simulink model "SG_RaibertControlMonopod"  (R2022a)
settings: Solver=ode4  StartTime=0.0  StopTime=inf  FixedStep=1/4000  MaxStep=0.001  RelTol=1e-3  AbsTol=1e-3  EnableMultiTasking=on
values from neighbouring files (symbols this model uses):
  alternate_legs = InitConstants.alternate_legs    [Controller.m]    (also in ControllerV2.m; ControllerV3.m; Controller_original.m; initialization.m = 1)
  dphi_IC = InitConstants.dphi_IC    [Controller.m]    (also in ControllerV2.m; ControllerV3.m; Controller_original.m; initialization.m = 0)
  dphi_RC_14 = 0.0    (= 0)    [initialization.m]
  dphi_RC_23 = 0.0    (= 0)    [initialization.m]
  dr_contact = -0.2    [initialization.m]
  dr_IC = InitConstants.dr_IC    [Controller.m]    (also in ControllerV2.m; ControllerV3.m; Controller_original.m; initialization.m = 0)
  dr_RC_14 = 0.0    (= 0)    [initialization.m]
  dr_RC_23 = 0.0    (= 0)    [initialization.m]
  dx_des = -InitConstants.dx_des    [Controller.m]    (also in ControllerV2.m; ControllerV3.m; Controller_original.m; Hopper_raibert_controller.m = -min(max(1.0*(x_body - x_des), -0.5), 0.5))
  Fthrust_RC_14 = 100    [initialization.m]
  Fthrust_RC_23 = 150    [initialization.m]
  GAIN_dx_RC_14 = 0.07    [initialization.m]
  GAIN_dx_RC_23 = 0.05    [initialization.m]
  Kd_phi_IC = InitConstants.Kd_phi_IC    [Controller.m]    (also in ControllerV2.m; ControllerV3.m; Controller_original.m; initialization.m = 15)
  Kd_phi_RC_14 = Kp_phi_RC_14*0.1    (= 10)    [initialization.m]
  Kd_phi_RC_23 = 15    [initialization.m]
  Kd_r_IC = InitConstants.Kd_r_IC    [Controller.m]    (also in ControllerV2.m; ControllerV3.m; Controller_original.m; initialization.m = 60)
  Kd_r_RC_14 = Kp_r_RC_14*0.1    (= 60)    [initialization.m]
  Kd_r_RC_23 = 150    [initialization.m]
  knee_limit = 160    [initialization.m]
  Kp_phi_IC = InitConstants.Kp_phi_IC    [Controller.m]    (also in ControllerV2.m; ControllerV3.m; Controller_original.m; initialization.m = 100)
  Kp_phi_RC_14 = 100    [initialization.m]
  Kp_phi_RC_23 = 100    [initialization.m]
  Kp_r_IC = InitConstants.Kp_r_IC    [Controller.m]    (also in ControllerV2.m; ControllerV3.m; Controller_original.m; initialization.m = 500)
  Kp_r_RC_14 = 600    [initialization.m]
  Kp_r_RC_23 = 600    [initialization.m]
  m_eff = 5    [ControllerV2.m]    (also in Controller_original.m; initialization.m)
  match_leg_gains = -1    [initialization.m]
  offset_phi_limit = 30    [initialization.m]
  phi_IC = InitConstants.phi_IC    [Controller.m]    (also in ControllerV2.m; ControllerV3.m; Controller_original.m; initialization.m = 0)
  phi_RC_14 = -0.003    [initialization.m]
  phi_RC_23 = -0.006    [initialization.m]
  r_IC = InitConstants.r_IC    [Controller.m]    (also in ControllerV2.m; ControllerV3.m; Controller_original.m; initialization.m = 0.32)
  r_RC_14 = 0.32    [initialization.m]
  r_RC_23 = 0.33    [initialization.m]
  r_thrust_RC_14 = 0.27    [initialization.m]
  r_thrust_RC_23 = 0.29    [initialization.m]
  tau_limit = 100    [initialization.m]
  update_controller_Kd_r = 1    [initialization.m]
  x_des = InitConstants.x_des    [Controller.m]    (also in ControllerV2.m; ControllerV3.m; Controller_original.m; initialization.m = 0)
undefined symbols (not defined in the file or in its folder): HS, IO291
libraries: speedgoatlib_IO691 x7, canmsglib x5, aru_toolbox x2, simulink x2, speedgoatlib_IO291 x1
(part 1 of 2)
settings Model: Creator=user  LastModifiedBy=Mechatronics
settings SolverCC: AutoScaleAbsTol=off  ConcurrentTasks=on  ZeroCrossAlgorithm=Adaptive  PositivePriorityOrder=on  AutoInsertRateTranBlk=on  MaxZcPerStep=1
settings DataIOCC: LimitDataPoints=on  MaxDataPoints=10000
settings OptimizationCC: BlockReduction=off  OptimizeBlockIOStorage=off
settings DebuggingCC: TasksWithSamePriorityMsg=none  UnconnectedInputMsg=warning  UnconnectedOutputMsg=warning  UnconnectedLineMsg=warning  AllowSymbolicDim=off  SFUnexpectedBacktrackingDiag=warning  SFNoUnconditionalDefaultTransitionDiag=warning  SFExecutionAtInitializationDiag=none  SFMachineParentedDataDiag=warning  ArithmeticOperatorsInVariantConditions=warning
settings HardwareCC: ProdBitPerLong=64  ProdLongLongMode=on  ProdHWDeviceType=Intel->x86-64 (Linux 64)
settings SFSimCC: SimUseLocalCustomCode=off  CustomCodeUndefinedFunction=UseInterfaceOnly
settings RTWCC: Description=Simulink Real-Time  SystemTargetFile=slrealtime.tlc  TemplateMakefile=slrealtime_default_tmf  RTWUseLocalCustomCode=off  Toolchain=Simulink Real-Time Toolchain  BuildConfiguration=Faster Runs  CodeExecutionProfiling=on  TargetLang=C++  DLArmComputeVersion=19.05
settings CodeAppCC: StateflowObjectComments=on
settings ConfigComp: CovMetricSettings=dw  CovSaveCumulativeToWorkspaceVar=on  CovSaveSingleToWorkspaceVar=on  CovExternalEMLEnable=off  CovSFcnEnable=off
settings SimscapeCC: SimscapeLogType=all  SimscapeLogSimulationStatistics=on  SimscapeLogDataHistory=10000
settings ExplorerConfigSet: InternalSimMechanicsExplorerSettings="<ExplorerConfiguration><canonicalview>planar_xy</canonicalview><AnimationSetting><BasePlaybackSpeed>1.0</BasePlaybackSpeed><PlaybackSpeedFactor>0.5</PlaybackSpeedFactor></AnimationSetting><TilePanel><TileInfo><Tiles Columns=\"1\" Count=\"1\" Rows=\"1\"><Column Weight=\"1\"/><Row Weight=\"1\"/><Tile Height=\"1\" Width=\"1\" X=\"0\" Y=\"0\"/></Tiles></TileInfo><SceneInfo><SceneViewer><BGColor><R>0.60000002384185791</R><G>0.60000002384185791</G><B>0.60000002384185791</B></BGColor><Camera><DoPerspective>off</DoPerspective><Position><X>-1.75490981765257059</X><Y>-0.0773030896581384797</Y><Z>0.0348947486595036771</Z></Position><Center><X>0.999999770911101038</X><Y>-0.0773030896581384797</Y><Z>0.0348947486595036771</Z></Center><Up><X>-0</X><Y>1</Y><Z>0</Z></Up><ViewLimDist>1</ViewLimDist><YLim>1.12613649771734692</YLim><XLim>1.72330216917466328</XLim></Camera></SceneViewer></SceneInfo></TilePanel><MechEditorPanel><Cameras/><GfxPanelCameraMap/><VideoCreator><PlaybackSpeedRatio>1.0</PlaybackSpeedRatio><FrameRate>30</FrameRate><VideoFormat>Motion JPEG AVI</VideoFormat><FrameSize>auto</FrameSize></VideoCreator></MechEditorPanel></ExplorerConfiguration>"

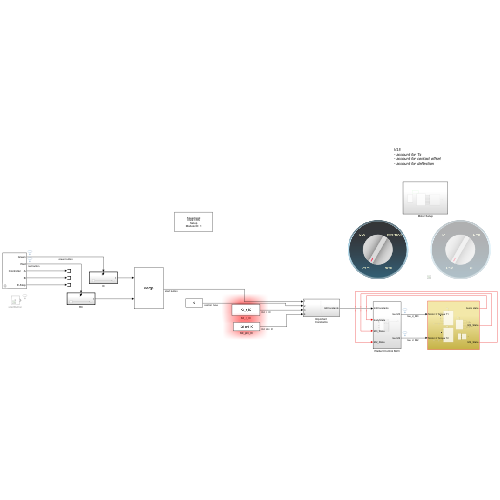
[thumbnail: Simulink's stored preview of the top-level diagram]
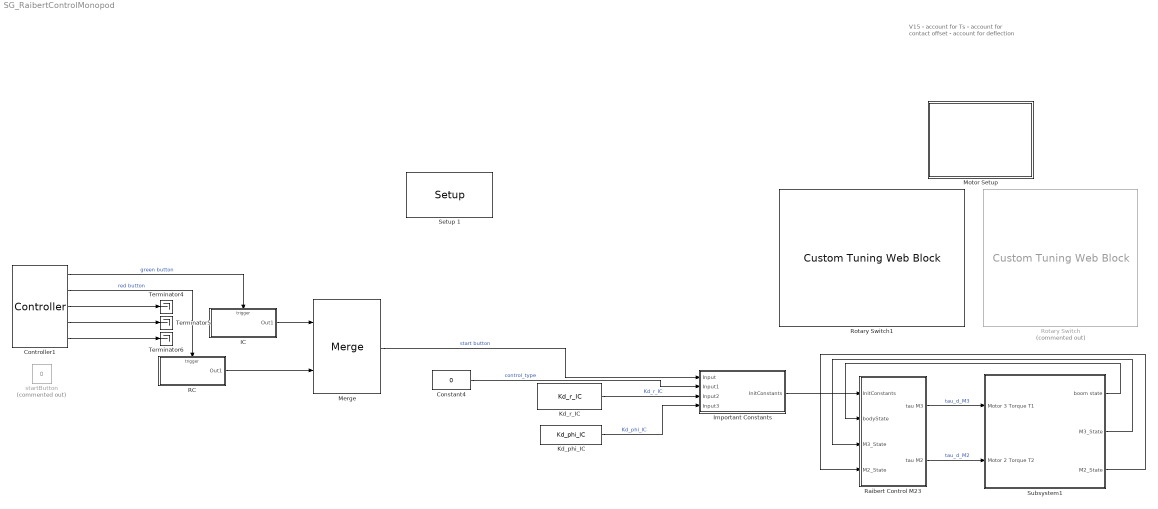
== system SG_RaibertControlMonopod ==
  note: V15
      | - account for Ts
      | - account for contact offset
      | - account for deflection
  Constant4 : Constant  Value=0
  Controller1 : aru_toolbox/Controller
      settings: SourceProductName=ARU Toolbox
  IC : Subsystem  TreatAsAtomicUnit=on
  Important Constants : Subsystem
  Kd_phi_IC : Constant  Value=Kd_phi_IC
  Kd_r_IC : Constant  Value=Kd_r_IC
  Merge : Merge  InitialOutput=[0]
  Motor Setup : Subsystem
  RC : Subsystem  TreatAsAtomicUnit=on
  Raibert Control M23 : Subsystem
  Rotary Switch : CustomTuningWebBlock  Commented=on  LabelPosition=Hide  ShowInitialText=on  Configuration="{\"components\":[{\"name\":\"RotarySwitchComponent\",\"settings\":{\"arcAngle\":300,\"arcAngleOffset\":120,\"handle\":{\"size\":[150,150],\"src\":\"data:image\\/svg+xml;base64,PHN2ZyBpZD0iTGF5ZXJfMSIgZGF0YS1uYW1lPSJMYXllciAxIiB4bWxucz0iaHR0cDovL3d3dy53My5vcmcvMjAwMC9zdmciIHhtbG5zOnhsaW5rPSJodHRwOi8vd3d3LnczLm9yZy8xOTk5L3hsaW5rIiB2aWV3Qm94PSIwIDAgMTIxIDEyMSI+PGRlZnM+PHN0eWxlPi5jbHMtMXtmaWxsOnVybCgjbGluZWFyLWdyYWRpZW50KTt9LmNscy0yLC5jbHMtM3tmaWxsOiNkMWQxZDE7fS5jbHMtM3tzdHJva2U6I2I3YjdiNztzdHJva2UtbWl0ZXJsaW1pdDoxMDtzdHJva2Utd2lkdGg6MC4yNXB4O30uY2xzLTR7ZmlsbDojZjMwMDAwO30uY2xzLTV7ZmlsbDojZjIxNzY3O308L3N0eWxlPjxsaW5lYXJHcmFkaWVudCBpZD0ibGluZWFyLWdyYWRpZW50IiB4MT0iNjAuNSIgeTE9IjEyMC41IiB4Mj0iNjAuNSIgeTI9IjAuNSIgZ3JhZGllbnRVbml0cz0idXNlclNwYWNlT25Vc2UiPjxzdG9wIG9mZnNldD0iMCIgc3RvcC1jb2xvcj0iI2QxZDFkMSIvPjxzdG9wIG9mZnNldD0iMC4xIiBzdG9wLWNvbG9yPSIjY2VjZWNlIi8+PHN0b3Agb2Zmc2V0PSIwLjE5IiBzdG9wLWNvbG9yPSIjYzNjM2MzIi8+PHN0b3Agb2Zmc2V0PSIwLjI4IiBzdG9wLWNvbG9yPSIjYjFiMWIxIi8+PHN0b3Agb2Zmc2V0PSIwLjM2IiBzdG9wLWNvbG9yPSIjOTg5ODk4Ii8+PHN0b3Agb2Zmc2V0PSIwLjQ0IiBzdG9wLWNvbG9yPSIjNzg3ODc4Ii8+PHN0b3Agb2Zmc2V0PSIwLjQ2IiBzdG9wLWNvbG9yPSIjNmI2YjZiIi8+PHN0b3Agb2Zmc2V0PSIwLjU0IiBzdG9wLWNvbG9yPSIjNmI2YjZiIi8+PHN0b3Agb2Zmc2V0PSIwLjU2IiBzdG9wLWNvbG9yPSIjNzY3Njc2Ii8+PHN0b3Agb2Zmc2V0PSIwLjY0IiBzdG9wLWNvbG9yPSIjOTc5Nzk3Ii8+PHN0b3Agb2Zmc2V0PSIwLjcyIiBzdG9wLWNvbG9yPSIjYjBiMGIwIi8+PHN0b3Agb2Zmc2V0PSIwLjgxIiBzdG9wLWNvbG9yPSIjYzNjM2MzIi8+PHN0b3Agb2Zmc2V0PSIwLjkiIHN0b3AtY29sb3I9IiNjZGNkY2QiLz48c3RvcCBvZmZzZXQ9IjEiIHN0b3AtY29sb3I9IiNkMWQxZDEiLz48L2xpbmVhckdyYWRpZW50PjwvZGVmcz48Y2lyY2xlIGNsYXNzPSJjbHMtMSIgY3g9IjYwLjUiIGN5PSI2MC41IiByPSI2MCIvPjxwYXRoIGNsYXNzPSJjbHMtMiIgZD0iTTYwLjUsMUE1OS41LDU5LjUsMCwxLDEsMSw2MC41LDU5LjU3LDU5LjU3LDAsMCwxLDYwLjUsMW0wLTFBNjAuNSw2MC41LDAsMSwwLDEyMSw2MC41LDYwLjUsNjAuNSwwLDAsMCw2MC41LDBaIi8+PHJlY3QgY2xhc3M9ImNscy0zIiB4PSIwLjUiIHk9IjUxLjUiIHdpZHRoPSIxMjAiIGhlaWdodD0iMTgiIHJ4PSIzLjA0Ii8+PHJlY3QgY2xhc3M9ImNscy00IiB4PSI1Ljc1IiB5PSI1OC43NSIgd2lkdGg9IjE2IiBoZWlnaHQ9IjMiLz48cGF0aCBjbGFzcz0iY2xzLTUiIGQ9Ik0yMS4yNSw1OS4yNXYyaC0xNXYtMmgxNW0xLTFoLTE3djRoMTd2LTRaIi8+PC9zdmc+\"},\"handleOffset\":[0,0],\"handleOrientation\":180,\"handlePosition\":[0,0,1,1],\"handleSize\":{\"height\":0.5,\"width\":0.5},\"labelRadius\":0.36,\"position\":[0,0,1,1],\"states\":[{\"Label\":{\"color\":[0,0,0,1],\"icon\":{\"size\":[0,0],\"src\":[],\"srcOrientation\":\"Right\"},\"iconPlacement\":\"left\",\"opacity\":1,\"position\":[0.7345552884615385,0.6796274038461538],\"show\":true,\"text\":{\"content\":\"Rest\",\"font\":\"Helvetica\",\"fontSize\":24}},\"Value\":0},{\"Label\":{\"color\":[0,0,0,1],\"icon\":{\"size\":[0,0],\"src\":[],\"srcOrientation\":\"Right\"},\"iconPlacement\":\"left\",\"opacity\":1,\"position\":[0.35757211538461536,0.7603966346153846],\"show\":true,\"text\":{\"content\":\"IC\",\"font\":\"Helvetica\",\"fontSize\":24}},\"Value\":1},{\"Label\":{\"color\":[0,0,0,1],\"icon\":{\"size\":[0,0],\"src\":[],\"srcOrientation\":\"Right\"},\"iconPlacement\":\"left\",\"opacity\":1,\"position\":[0.09603365384615385,0.46033653846153844],\"show\":true,\"text\":{\"content\":\"HOP\",\"font\":\"Helvetica\",\"fontSize\":24}},\"Value\":2},{\"Label\":{\"color\":[0,0,0],\"icon\":{\"size\":[1,1],\"src\":\"default\",\"srcOrientation\":\"Right\"},\"iconPlacement\":\"left\",\"opacity\":1,\"position\":[0,0],\"show\":true,\"text\":{\"content\":\"RC\",\"fontSize\":14}},\"Value\":3}],\"tickRadius\":0.32}},{\"name\":\"BackgroundImageComponent\",\"settings\":{\"image\":{\"size\":[155,150],\"src\":\"data:image\\/svg+xml;base64,PD94bWwgdmVyc2lvbj0iMS4wIiBlbmNvZGluZz0idXRmLTgiPz4NCjwhLS0gR2VuZXJhdG9yOiBBZG9iZSBJbGx1c3RyYXRvciAyNS4wLjAsIFNWRyBFeHBvcnQgUGx1Zy1JbiAuIFNWRyBWZXJzaW9uOiA2LjAwIEJ1aWxkIDApICAtLT4NCjxzdmcgdmVyc2lvbj0iMS4xIg0KCSBpZD0iTGF5ZXJfMl8xXyIgeG1sbnM6Y2M9Imh0dHA6Ly9jcmVhdGl2ZWNvbW1vbnMub3JnL25zIyIgeG1sbnM6ZGM9Imh0dHA6Ly9wdXJsLm9yZy9kYy9lbGVtZW50cy8xLjEvIiB4bWxuczppbmtzY2FwZT0iaHR0cDovL3d3dy5pbmtzY2FwZS5vcmcv ...(+4184 chars)\",\"srcOrientation\":\"Right\"},\"position\":[0,0,1,1],\"scaleMode\":\"0\"}},{\"name\":\"ForegroundImageComponent\",\"settings\":{\"image\":{\"size\":[0,0],\"src\":\"default\",\"srcOrientation\":[]},\"isForeground\":1,\"position\":[0,0,1,1],\"scaleMode\":\"0\"}}],\"settings\":{\"BindingType\":\"param\",\"backgroundColor\":[0,0,255,\"1\"],\"enumDataType\":\"\",\"fixedAspectRatio\":\"off\",\"image\":{\"size\":[150,150],\"src\":\"data:image\\/svg+xml;base64,PD94bWwgdmVyc2lvbj0iMS4wIiBlbmNvZGluZz0iVVRGLTgiIHN0YW5kYWxvbmU9Im5vIj8+CjwhLS0gR2VuZXJhdG9yOiBBZG9iZSBJbGx1c3RyYXRvciAxOS4yLjEsIFNWRyBFeHBvcnQgUGx1Zy1JbiAuIFNWRyBWZXJzaW9uOiA2LjAwIEJ1aWxkIDApICAtLT4KCjxzdmcKICAgeG1sbnM6ZGM9Imh0dHA6Ly9wdXJsLm9yZy9kYy9lbGVtZW50cy8xLjEvIgogICB4bWxuczpjYz0iaHR0cDovL2NyZWF0aXZlY29tbW9ucy5vcmcvbnMjIgogICB4bWxuczpyZGY9Imh0dHA6Ly93d3cudzMub3JnLzE5OTkvMDIvMjItcmRmLXN5bnRh ...(+9660 chars)\"},\"showBackgroundColor\":false,\"useEnumDataType\":false,\"variant\":\"rotarySwitch\"},\"type\":\"RotarySwitch\"}"
  Rotary Switch1 : CustomTuningWebBlock  LabelPosition=Hide  ShowInitialText=on  Configuration="{\"components\":[{\"name\":\"RotarySwitchComponent\",\"settings\":{\"arcAngle\":300,\"arcAngleOffset\":120,\"handle\":{\"size\":[150,150],\"src\":\"data:image\\/svg+xml;base64,PHN2ZyBpZD0iTGF5ZXJfMSIgZGF0YS1uYW1lPSJMYXllciAxIiB4bWxucz0iaHR0cDovL3d3dy53My5vcmcvMjAwMC9zdmciIHhtbG5zOnhsaW5rPSJodHRwOi8vd3d3LnczLm9yZy8xOTk5L3hsaW5rIiB2aWV3Qm94PSIwIDAgMTIxIDEyMSI+PGRlZnM+PHN0eWxlPi5jbHMtMXtmaWxsOnVybCgjbGluZWFyLWdyYWRpZW50KTt9LmNscy0yLC5jbHMtM3tmaWxsOiNkMWQxZDE7fS5jbHMtM3tzdHJva2U6I2I3YjdiNztzdHJva2UtbWl0ZXJsaW1pdDoxMDtzdHJva2Utd2lkdGg6MC4yNXB4O30uY2xzLTR7ZmlsbDojZjMwMDAwO30uY2xzLTV7ZmlsbDojZjIxNzY3O308L3N0eWxlPjxsaW5lYXJHcmFkaWVudCBpZD0ibGluZWFyLWdyYWRpZW50IiB4MT0iNjAuNSIgeTE9IjEyMC41IiB4Mj0iNjAuNSIgeTI9IjAuNSIgZ3JhZGllbnRVbml0cz0idXNlclNwYWNlT25Vc2UiPjxzdG9wIG9mZnNldD0iMCIgc3RvcC1jb2xvcj0iI2QxZDFkMSIvPjxzdG9wIG9mZnNldD0iMC4xIiBzdG9wLWNvbG9yPSIjY2VjZWNlIi8+PHN0b3Agb2Zmc2V0PSIwLjE5IiBzdG9wLWNvbG9yPSIjYzNjM2MzIi8+PHN0b3Agb2Zmc2V0PSIwLjI4IiBzdG9wLWNvbG9yPSIjYjFiMWIxIi8+PHN0b3Agb2Zmc2V0PSIwLjM2IiBzdG9wLWNvbG9yPSIjOTg5ODk4Ii8+PHN0b3Agb2Zmc2V0PSIwLjQ0IiBzdG9wLWNvbG9yPSIjNzg3ODc4Ii8+PHN0b3Agb2Zmc2V0PSIwLjQ2IiBzdG9wLWNvbG9yPSIjNmI2YjZiIi8+PHN0b3Agb2Zmc2V0PSIwLjU0IiBzdG9wLWNvbG9yPSIjNmI2YjZiIi8+PHN0b3Agb2Zmc2V0PSIwLjU2IiBzdG9wLWNvbG9yPSIjNzY3Njc2Ii8+PHN0b3Agb2Zmc2V0PSIwLjY0IiBzdG9wLWNvbG9yPSIjOTc5Nzk3Ii8+PHN0b3Agb2Zmc2V0PSIwLjcyIiBzdG9wLWNvbG9yPSIjYjBiMGIwIi8+PHN0b3Agb2Zmc2V0PSIwLjgxIiBzdG9wLWNvbG9yPSIjYzNjM2MzIi8+PHN0b3Agb2Zmc2V0PSIwLjkiIHN0b3AtY29sb3I9IiNjZGNkY2QiLz48c3RvcCBvZmZzZXQ9IjEiIHN0b3AtY29sb3I9IiNkMWQxZDEiLz48L2xpbmVhckdyYWRpZW50PjwvZGVmcz48Y2lyY2xlIGNsYXNzPSJjbHMtMSIgY3g9IjYwLjUiIGN5PSI2MC41IiByPSI2MCIvPjxwYXRoIGNsYXNzPSJjbHMtMiIgZD0iTTYwLjUsMUE1OS41LDU5LjUsMCwxLDEsMSw2MC41LDU5LjU3LDU5LjU3LDAsMCwxLDYwLjUsMW0wLTFBNjAuNSw2MC41LDAsMSwwLDEyMSw2MC41LDYwLjUsNjAuNSwwLDAsMCw2MC41LDBaIi8+PHJlY3QgY2xhc3M9ImNscy0zIiB4PSIwLjUiIHk9IjUxLjUiIHdpZHRoPSIxMjAiIGhlaWdodD0iMTgiIHJ4PSIzLjA0Ii8+PHJlY3QgY2xhc3M9ImNscy00IiB4PSI1Ljc1IiB5PSI1OC43NSIgd2lkdGg9IjE2IiBoZWlnaHQ9IjMiLz48cGF0aCBjbGFzcz0iY2xzLTUiIGQ9Ik0yMS4yNSw1OS4yNXYyaC0xNXYtMmgxNW0xLTFoLTE3djRoMTd2LTRaIi8+PC9zdmc+\"},\"handleOffset\":[0,0],\"handleOrientation\":180,\"handlePosition\":[0,0,1,1],\"handleSize\":{\"height\":0.5,\"width\":0.5},\"labelRadius\":0.36,\"position\":[0,0,1,1],\"states\":[{\"Label\":{\"color\":[0,0,0,1],\"icon\":{\"size\":[0,0],\"src\":[],\"srcOrientation\":\"Right\"},\"iconPlacement\":\"left\",\"opacity\":1,\"position\":[0.7345552884615385,0.6796274038461538],\"show\":true,\"text\":{\"content\":\"dx = 0\",\"font\":\"Helvetica\",\"fontSize\":24}},\"Value\":0},{\"Label\":{\"color\":[0,0,0,1],\"icon\":{\"size\":[0,0],\"src\":[],\"srcOrientation\":\"Right\"},\"iconPlacement\":\"left\",\"opacity\":1,\"position\":[0.35757211538461536,0.7603966346153846],\"show\":true,\"text\":{\"content\":\"dx>0\",\"font\":\"Helvetica\",\"fontSize\":24}},\"Value\":1},{\"Label\":{\"color\":[0,0,0,1],\"icon\":{\"size\":[0,0],\"src\":[],\"srcOrientation\":\"Right\"},\"iconPlacement\":\"left\",\"opacity\":1,\"position\":[0.09603365384615385,0.46033653846153844],\"show\":true,\"text\":{\"content\":\"POSITION\",\"font\":\"Helvetica\",\"fontSize\":24}},\"Value\":2},{\"Label\":{\"color\":[0,0,0],\"icon\":{\"size\":[1,1],\"src\":\"default\",\"srcOrientation\":\"Right\"},\"iconPlacement\":\"left\",\"opacity\":1,\"position\":[0,0],\"show\":true,\"text\":{\"content\":\"dx<0\",\"fontSize\":14}},\"Value\":3}],\"tickRadius\":0.32}},{\"name\":\"BackgroundImageComponent\",\"settings\":{\"image\":{\"size\":[155,150],\"src\":\"data:image\\/svg+xml;base64,PD94bWwgdmVyc2lvbj0iMS4wIiBlbmNvZGluZz0idXRmLTgiPz4NCjwhLS0gR2VuZXJhdG9yOiBBZG9iZSBJbGx1c3RyYXRvciAyNS4wLjAsIFNWRyBFeHBvcnQgUGx1Zy1JbiAuIFNWRyBWZXJzaW9uOiA2LjAwIEJ1aWxkIDApICAtLT4NCjxzdmcgdmVyc2lvbj0iMS4xIg0KCSBpZD0iTGF5ZXJfMl8xXyIgeG1sbnM6Y2M9Imh0dHA6Ly9jcmVhdGl2ZWNvbW1vbnMub3JnL25zIyIgeG1sbnM6ZGM9Imh0dHA6Ly9wdXJsLm9yZy9kYy9lbGVtZW50cy8xLjEvIiB4bWxuczppbmtzY2FwZT0iaHR0cDovL3d3dy5pbmtzY2FwZS5vcmcv ...(+4184 chars)\",\"srcOrientation\":\"Right\"},\"position\":[0,0,1,1],\"scaleMode\":\"0\"}},{\"name\":\"ForegroundImageComponent\",\"settings\":{\"image\":{\"size\":[0,0],\"src\":\"default\",\"srcOrientation\":[]},\"isForeground\":1,\"position\":[0,0,1,1],\"scaleMode\":\"0\"}}],\"settings\":{\"BindingType\":\"param\",\"backgroundColor\":[0,0,255,\"1\"],\"enumDataType\":\"\",\"fixedAspectRatio\":\"off\",\"image\":{\"size\":[150,150],\"src\":\"data:image\\/svg+xml;base64,PD94bWwgdmVyc2lvbj0iMS4wIiBlbmNvZGluZz0iVVRGLTgiIHN0YW5kYWxvbmU9Im5vIj8+CjwhLS0gR2VuZXJhdG9yOiBBZG9iZSBJbGx1c3RyYXRvciAxOS4yLjEsIFNWRyBFeHBvcnQgUGx1Zy1JbiAuIFNWRyBWZXJzaW9uOiA2LjAwIEJ1aWxkIDApICAtLT4KCjxzdmcKICAgeG1sbnM6ZGM9Imh0dHA6Ly9wdXJsLm9yZy9kYy9lbGVtZW50cy8xLjEvIgogICB4bWxuczpjYz0iaHR0cDovL2NyZWF0aXZlY29tbW9ucy5vcmcvbnMjIgogICB4bWxuczpyZGY9Imh0dHA6Ly93d3cudzMub3JnLzE5OTkvMDIvMjItcmRmLXN5bnRh ...(+9660 chars)\"},\"showBackgroundColor\":false,\"useEnumDataType\":false,\"variant\":\"rotarySwitch\"},\"type\":\"RotarySwitch\"}"
  Setup 1 : speedgoatlib_IO291/Setup   parInternalModuleId=1  parPciSlot=-1  parModuleId=1  parModuleType=IO291-HS  parTtlDoChannels=[]  parTtlDoInitValues=1  parTtlDoReset=1  parTtlDiChannels=[1 2 3 4 5]  parIsolDiChannels=[]  parFetDoChannels=[]  parFetDoInitValues=0  parFetDoReset=0
      settings: SourceProductName=Simulink Real-Time: Speedgoat I/O Blockset
  Subsystem1 : Subsystem
  Terminator4 : Terminator
  Terminator5 : Terminator
  Terminator6 : Terminator
  startButton : Constant  Commented=on  Value=0
  wires:
  Controller1/1 -> IC/Trigger  "green button"
  Controller1/5 -> Terminator6/1
  Controller1/3 -> Terminator4/1
  Controller1/4 -> Terminator5/1
  Important Constants/1(InitConstants) -> Raibert Control M23/1(InitConstants)
  Subsystem1/3(M2_State) -> Raibert Control M23/4(M2_State)
  Subsystem1/2(M3_State) -> Raibert Control M23/3(M3_State)
  Subsystem1/1(boom state) -> Raibert Control M23/2(bodyState)
  Raibert Control M23/1(tau M3) -> Subsystem1/1(Motor 3 Torque T1)  "tau_d_M3"
  Raibert Control M23/2(tau M2) -> Subsystem1/2(Motor 2 Torque T2)  "tau_d_M2"
  Merge/1 -> Important Constants/1(Input)  "start button"
  Constant4/1 -> Important Constants/2(Input1)  "control_type"
  Kd_r_IC/1 -> Important Constants/3(Input2)  "Kd_r_IC"
  Kd_phi_IC/1 -> Important Constants/4(Input3)  "Kd_phi_IC"
  Controller1/2 -> RC/Trigger  "red button"
  RC/1(Out1) -> Merge/2
  IC/1(Out1) -> Merge/1

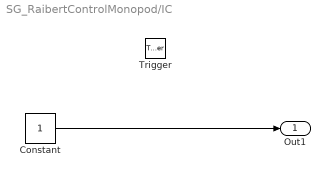
== system SG_RaibertControlMonopod/IC ==
  Trigger : TriggerPort  VariantControl=(inherit)
  Constant : Constant
  Out1 : Outport
  wires:
  Constant/1 -> Out1/1

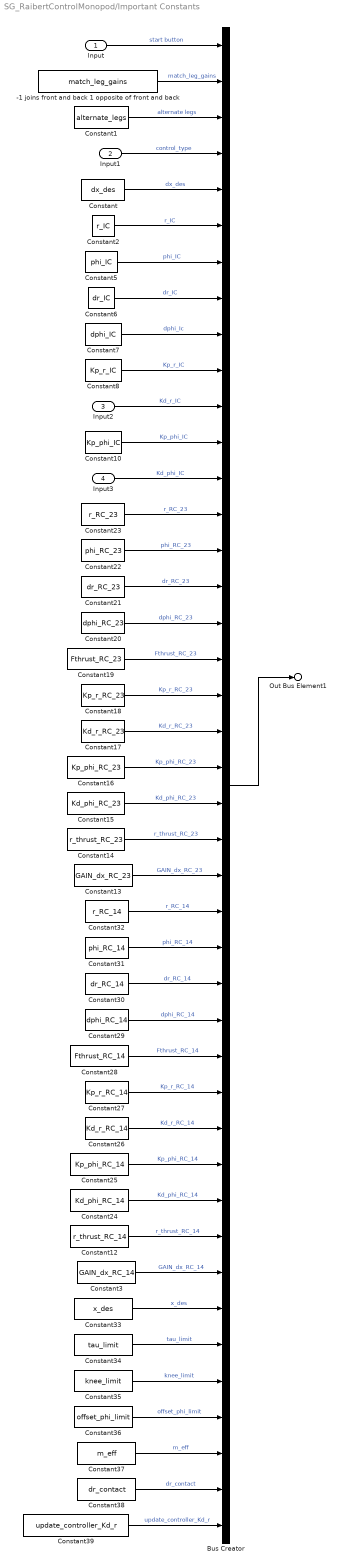
== system SG_RaibertControlMonopod/Important Constants ==
  Input : Inport
  Input1 : Inport  Port=2
  Input2 : Inport  Port=3
  Input3 : Inport  Port=4
  -1 joins front and back 1 opposite of front and back : Constant  Value=match_leg_gains
  Bus Creator : BusCreator  Inputs=42  OutDataTypeStr=Bus: InitConstants
  Constant : Constant  Value=dx_des
  Constant1 : Constant  Value=alternate_legs
  Constant10 : Constant  Value=Kp_phi_IC
  Constant12 : Constant  Value=r_thrust_RC_14
  Constant13 : Constant  Value=GAIN_dx_RC_23
  Constant14 : Constant  Value=r_thrust_RC_23
  Constant15 : Constant  Value=Kd_phi_RC_23
  Constant16 : Constant  Value=Kp_phi_RC_23
  Constant17 : Constant  Value=Kd_r_RC_23
  Constant18 : Constant  Value=Kp_r_RC_23
  Constant19 : Constant  Value=Fthrust_RC_23
  Constant2 : Constant  Value=r_IC
  Constant20 : Constant  Value=dphi_RC_23
  Constant21 : Constant  Value=dr_RC_23
  Constant22 : Constant  Value=phi_RC_23
  Constant23 : Constant  Value=r_RC_23
  Constant24 : Constant  Value=Kd_phi_RC_14
  Constant25 : Constant  Value=Kp_phi_RC_14
  Constant26 : Constant  Value=Kd_r_RC_14
  Constant27 : Constant  Value=Kp_r_RC_14
  Constant28 : Constant  Value=Fthrust_RC_14
  Constant29 : Constant  Value=dphi_RC_14
  Constant3 : Constant  Value=GAIN_dx_RC_14
  Constant30 : Constant  Value=dr_RC_14
  Constant31 : Constant  Value=phi_RC_14
  Constant32 : Constant  Value=r_RC_14
  Constant33 : Constant  Value=x_des
  Constant34 : Constant  Value=tau_limit
  Constant35 : Constant  Value=knee_limit
  Constant36 : Constant  Value=offset_phi_limit
  Constant37 : Constant  Value=m_eff
  Constant38 : Constant  Value=dr_contact
  Constant39 : Constant  Value=update_controller_Kd_r
  Constant5 : Constant  Value=phi_IC
  Constant6 : Constant  Value=dr_IC
  Constant7 : Constant  Value=dphi_IC
  Constant8 : Constant  Value=Kp_r_IC
  Out Bus Element1 : Outport  VectorParamsAs1DForOutWhenUnconnected=off  PortName=InitConstants
  wires:
  -1 joins front and back 1 opposite of front and back/1 -> Bus Creator/2  "match_leg_gains"
  Input/1 -> Bus Creator/1  "start button"
  Constant/1 -> Bus Creator/5  "dx_des"
  Constant1/1 -> Bus Creator/3  "alternate legs"
  Input1/1 -> Bus Creator/4  "control_type"
  Constant2/1 -> Bus Creator/6  "r_IC"
  Constant5/1 -> Bus Creator/7  "phi_IC"
  Constant6/1 -> Bus Creator/8  "dr_IC"
  Constant7/1 -> Bus Creator/9  "dphi_Ic"
  Constant8/1 -> Bus Creator/10  "Kp_r_IC"
  Input2/1 -> Bus Creator/11  "Kd_r_IC"
  Constant10/1 -> Bus Creator/12  "Kp_phi_IC"
  Constant18/1 -> Bus Creator/19  "Kp_r_RC_23"
  Constant17/1 -> Bus Creator/20  "Kd_r_RC_23"
  Constant15/1 -> Bus Creator/22  "Kd_phi_RC_23"
  Constant21/1 -> Bus Creator/16  "dr_RC_23"
  Input3/1 -> Bus Creator/13  "Kd_phi_IC"
  Constant23/1 -> Bus Creator/14  "r_RC_23"
  Constant22/1 -> Bus Creator/15  "phi_RC_23"
  Constant20/1 -> Bus Creator/17  "dphi_RC_23"
  Constant19/1 -> Bus Creator/18  "Fthrust_RC_23"
  Constant13/1 -> Bus Creator/24  "GAIN_dx_RC_23"
  Constant14/1 -> Bus Creator/23  "r_thrust_RC_23"
  Constant16/1 -> Bus Creator/21  "Kp_phi_RC_23"
  Bus Creator/1 -> Out Bus Element1/1
  Constant33/1 -> Bus Creator/36  "x_des"
  Constant28/1 -> Bus Creator/29  "Fthrust_RC_14"
  Constant12/1 -> Bus Creator/34  "r_thrust_RC_14"
  Constant26/1 -> Bus Creator/31  "Kd_r_RC_14"
  Constant24/1 -> Bus Creator/33  "Kd_phi_RC_14"
  Constant29/1 -> Bus Creator/28  "dphi_RC_14"
  Constant31/1 -> Bus Creator/26  "phi_RC_14"
  Constant32/1 -> Bus Creator/25  "r_RC_14"
  Constant27/1 -> Bus Creator/30  "Kp_r_RC_14"
  Constant25/1 -> Bus Creator/32  "Kp_phi_RC_14"
  Constant3/1 -> Bus Creator/35  "GAIN_dx_RC_14"
  Constant30/1 -> Bus Creator/27  "dr_RC_14"
  Constant34/1 -> Bus Creator/37  "tau_limit"
  Constant35/1 -> Bus Creator/38  "knee_limit"
  Constant36/1 -> Bus Creator/39  "offset_phi_limit"
  Constant37/1 -> Bus Creator/40  "m_eff"
  Constant38/1 -> Bus Creator/41  "dr_contact"
  Constant39/1 -> Bus Creator/42  "update_controller_Kd_r"
